simulink model "verify_Pressure_Drop_changeD_mdl"  (R2016b)
settings: Solver=VariableStepDiscrete  StartTime=0.0  StopTime=10  MaxStep=1  RelTol=1e-3  EnableMultiTasking=on
undefined symbols (not defined in the file or in its folder): DiameterLastPiece, DPConstant, DPLinear, DPQuadratic, Pressure
libraries: carnot x6, simulink x1
settings Model: Creator=drhf  LastModifiedBy=drhf
settings DataIOCC: LimitDataPoints=on  SaveFormat=Array  SignalLoggingSaveFormat=ModelDataLogs
settings OptimizationCC: ExpressionDepthLimit=2147483647  LifeSpan=inf
settings DebuggingCC: UnderspecifiedInitializationDetection=Classic  MergeDetectMultiDrivingBlocksExec=none  SolverPrmCheckMsg=warning  FcnCallInpInsideContextMsg=warning  StateNameClashWarn=warning  SFUnexpectedBacktrackingDiag=warning  SFNoUnconditionalDefaultTransitionDiag=warning  SFExecutionAtInitializationDiag=none
settings HardwareCC: ProdBitPerPointer=32  ProdBitPerSizeT=32  ProdBitPerPtrDiffT=32  ProdLargestAtomicFloat=None  ProdIntDivRoundTo=Undefined  ProdEndianess=Unspecified  ProdWordSize=32  ProdHWDeviceType=32-bit Generic
settings ModelReferenceCC: PropagateSignalLabelsOutOfModel=off
settings GRTTargetCC: TargetLangStandard=C89/C90 (ANSI)  GeneratePreprocessorConditionals=Disable all  CombineOutputUpdateFcns=off  GRTInterface=on
settings ConfigComp: CovMetricSettings=dw  CovHtmlReporting=on  CovSaveCumulativeToWorkspaceVar=on  CovSaveSingleToWorkspaceVar=on  CovExternalEMLEnable=off

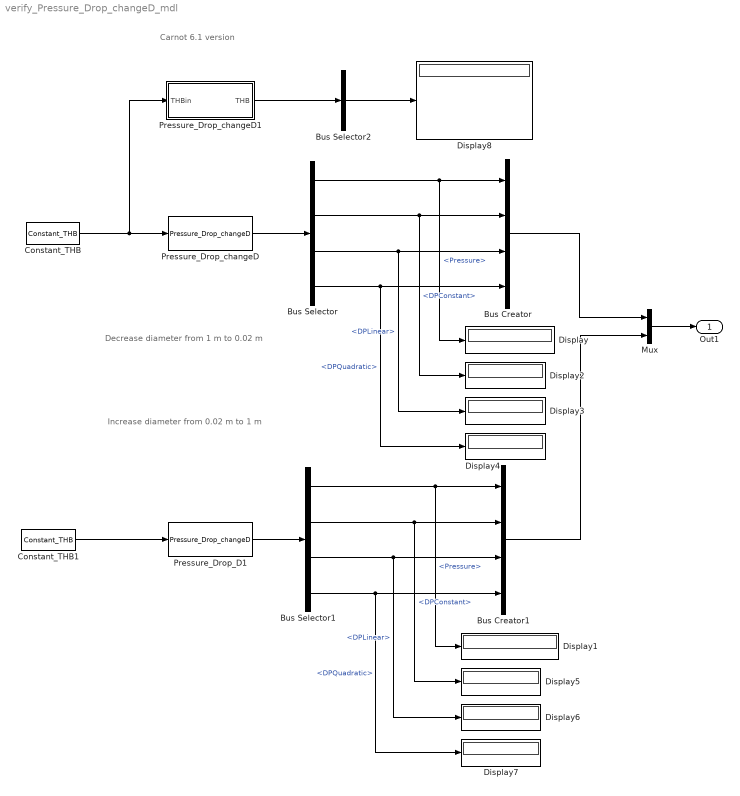
== system verify_Pressure_Drop_changeD_mdl ==
  note: Carnot 6.1 version
  note: Increase diameter from 0.02 m to 1 m
  note: Decrease diameter from 1 m to 0.02 m
  Bus Creator : BusCreator  Inputs=4
  Bus Creator1 : BusCreator  Inputs=4
  Bus Selector : BusSelector  OutputSignals=Pressure,DPConstant,DPLinear,DPQuadratic
  Bus Selector1 : BusSelector  OutputSignals=Pressure,DPConstant,DPLinear,DPQuadratic
  Bus Selector2 : BusSelector  OutputSignals=Pressure,DPConstant,DPLinear,DPQuadratic  OutputAsBus=on
  Constant_THB : carnot/Source/Simple/Constant_THB  t=40  mdot=100/3600  p=1e5  mID=Full Pressure Drop with Static Height  fluid=Water  mix=0  mix2=0  mix3=0  dia=1  hgt=0
  Constant_THB1 : carnot/Source/Simple/Constant_THB  t=40  mdot=100/3600  p=1e5  mID=Full Pressure Drop with Static Height  fluid=Water  mix=0  mix2=0  mix3=0  dia=0.02  hgt=0
  Display{,1..8} (9 alike) : Display
  Mux : Mux  Inputs=2
  Pressure_Drop_D1 : carnot/Basic/Pressure_Drop/Pressure_Drop_changeD  dia=1
  Pressure_Drop_changeD : carnot/Basic/Pressure_Drop/Pressure_Drop_changeD  dia=0.02
  Pressure_Drop_changeD1 : Subsystem  mask(Pressure Drop Change Diameter){dia=0.02}
      mask prompts: dia "Diameter in m"
      mask help: Calculates the pressure drop due to a diameter change at the inlet (of a pipe).
      mask Help: web(fullfile(path_carnot('help'),'Pressure_Drop_changeD.html'),'-helpbrowser')
  Out1 : Outport
  wires:
  Constant_THB/1 -> Pressure_Drop_changeD1/1(THBin), Pressure_Drop_changeD/1
  Pressure_Drop_changeD/1 -> Bus Selector/1
  Bus Selector/1 -> Display/1, Bus Creator/1  "<Pressure>"
  Bus Selector/2 -> Bus Creator/2, Display2/1  "<DPConstant>"
  Bus Selector/3 -> Bus Creator/3, Display3/1  "<DPLinear>"
  Bus Selector/4 -> Bus Creator/4, Display4/1  "<DPQuadratic>"
  Constant_THB1/1 -> Pressure_Drop_D1/1
  Pressure_Drop_D1/1 -> Bus Selector1/1
  Bus Selector1/1 -> Display1/1, Bus Creator1/1  "<Pressure>"
  Bus Selector1/2 -> Bus Creator1/2, Display5/1  "<DPConstant>"
  Bus Selector1/3 -> Bus Creator1/3, Display6/1  "<DPLinear>"
  Bus Selector1/4 -> Bus Creator1/4, Display7/1  "<DPQuadratic>"
  Mux/1 -> Out1/1
  Bus Creator/1 -> Mux/1
  Bus Creator1/1 -> Mux/2
  Pressure_Drop_changeD1/1(THB) -> Bus Selector2/1
  Bus Selector2/1 -> Display8/1

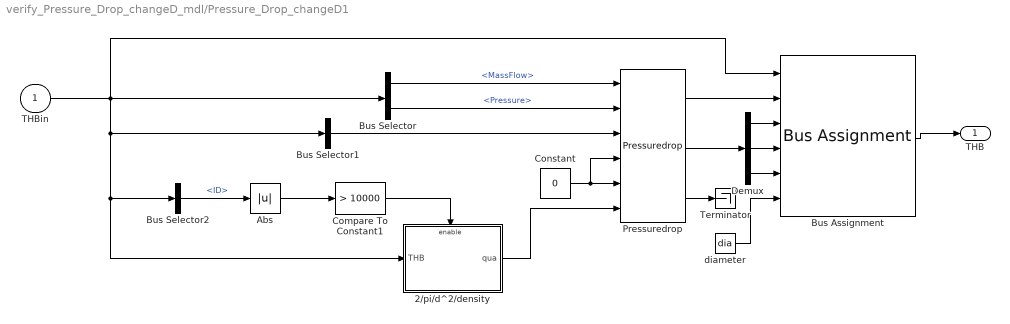
== system verify_Pressure_Drop_changeD_mdl/Pressure_Drop_changeD1 ==
  THBin : Inport
  2/pi/d^2/density : Subsystem
  Abs : Abs
  Bus Assignment : BusAssignment  AssignedSignals=Pressure,DPConstant,DPLinear,DPQuadratic,DiameterLastPiece
  Bus Selector : BusSelector  OutputSignals=MassFlow,Pressure
  Bus Selector1 : BusSelector  OutputSignals=DPConstant,DPLinear,DPQuadratic  OutputAsBus=on
  Bus Selector2 : BusSelector  OutputSignals=ID
  Compare To Constant1 : simulink/Logic and Bit Operations/Compare To Constant  relop=>  const=10000  OutDataTypeStr=boolean
  Constant : Constant  Value=0
  Demux : Demux  Outputs=3
  Pressuredrop : carnot/Basic/Pressure_Drop/Pressuredrop
  Terminator : Terminator
  diameter : Constant  Value=dia
  THB : Outport
  wires:
  Pressuredrop/3 -> Terminator/1
  Compare To Constant1/1 -> 2/pi/d^2/density/Enable
  2/pi/d^2/density/1(qua) -> Pressuredrop/6
  Constant/1 -> Pressuredrop/4, Pressuredrop/5
  Bus Selector2/1 -> Abs/1  "<ID>"
  Bus Selector/2 -> Pressuredrop/2  "<Pressure>"
  Bus Selector/1 -> Pressuredrop/1  "<MassFlow>"
  Bus Selector1/1 -> Pressuredrop/3
  Abs/1 -> Compare To Constant1/1
  THBin/1 -> 2/pi/d^2/density/1(THB), Bus Selector2/1, Bus Selector1/1, Bus Selector/1, Bus Assignment/1
  Bus Assignment/1 -> THB/1
  Pressuredrop/1 -> Bus Assignment/2
  Demux/1 -> Bus Assignment/3
  Demux/2 -> Bus Assignment/4
  Demux/3 -> Bus Assignment/5
  Pressuredrop/2 -> Demux/1
  diameter/1 -> Bus Assignment/6

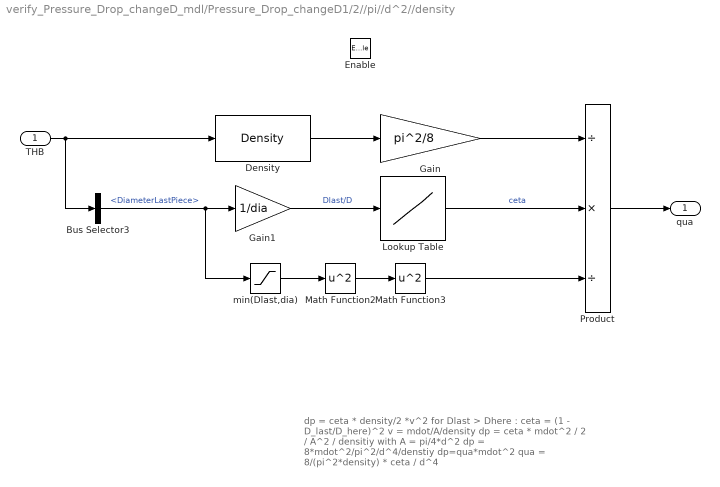
== system verify_Pressure_Drop_changeD_mdl/Pressure_Drop_changeD1/2//pi//d^2//density ==
  note: dp = ceta * density/2 *v^2
      | for Dlast > Dhere : ceta = (1 - D_last/D_here)^2
      | v = mdot/A/density
      | dp = ceta * mdot^2 / 2 / A^2 / densitiy
      | with A = pi/4*d^2
      | dp = 8*mdot^2/pi^2/d^4/denstiy
      | dp=qua*mdot^2
      | qua = 8/(pi^2*density) * ceta / d^4
  THB : Inport
  Enable : EnablePort
  Bus Selector3 : BusSelector  OutputSignals=DiameterLastPiece
  Density : carnot/Basic/Material_Properties/Density  VariantControl=CarlibClassic  INPUTARGUMENTS=THB  DEBUGLEVEL=DEBUGLEVEL  MAXTOTALWARNINGS=inf  MAXCONSECUTIVEWARNINGS=inf  WRITETOFILE=0  FILENAME='errors.txt'
  Gain : Gain  Gain=pi^2/8
  Gain1 : Gain  Gain=1/dia
  Lookup Table : Lookup  InputValues=[0:0.05:1, 10, 100]  Table="[(1 - [0:0.05:1]).^2,  1.2, 1.2]"
  Math Function2 : Math  Operator=square  SaturateOnIntegerOverflow=on
  Math Function3 : Math  Operator=square  SaturateOnIntegerOverflow=on
  Product : Product  Inputs=/*/  RndMeth=Zero
  min(Dlast,dia) : Saturate  UpperLimit=dia  LowerLimit=0
  qua : Outport
  wires:
  Lookup Table/1 -> Product/2  "ceta"
  Math Function3/1 -> Product/3
  Math Function2/1 -> Math Function3/1
  min(Dlast,dia)/1 -> Math Function2/1
  Gain1/1 -> Lookup Table/1  "Dlast/D"
  Product/1 -> qua/1
  Gain/1 -> Product/1
  Bus Selector3/1 -> min(Dlast,dia)/1, Gain1/1  "<DiameterLastPiece>"
  THB/1 -> Density/1, Bus Selector3/1
  Density/1 -> Gain/1
